simulink model "SUB_IoControl"  (R2018b)
settings: Solver=VariableStepDiscrete  StartTime=0.0  StopTime=10  RelTol=1e-3
PreLoadFcn:
  | if(exist('MBDS_ModelCallback', 'file'))
  |    MBDS_ModelCallback('PreLoad');
  | end
PostLoadFcn:
  | if(exist('MBDS_ModelCallback', 'file'))
  |    MBDS_ModelCallback('PostLoad');
  | end
InitFcn:
  | if(exist('MBDS_ModelCallback', 'file'))
  |    MBDS_ModelCallback('Init');
  | end
StartFcn:
  | if(exist('MBDS_ModelCallback', 'file'))
  |    MBDS_ModelCallback('Start');
  | end
StopFcn:
  | if(exist('MBDS_ModelCallback', 'file'))
  |    MBDS_ModelCallback('Stop');
  | end
undefined symbols (not defined in the file): sigbuilder_block
libraries: KIBES_Signal x742, MBDS_Modules x38, simulink x1
(part 8 of 8)

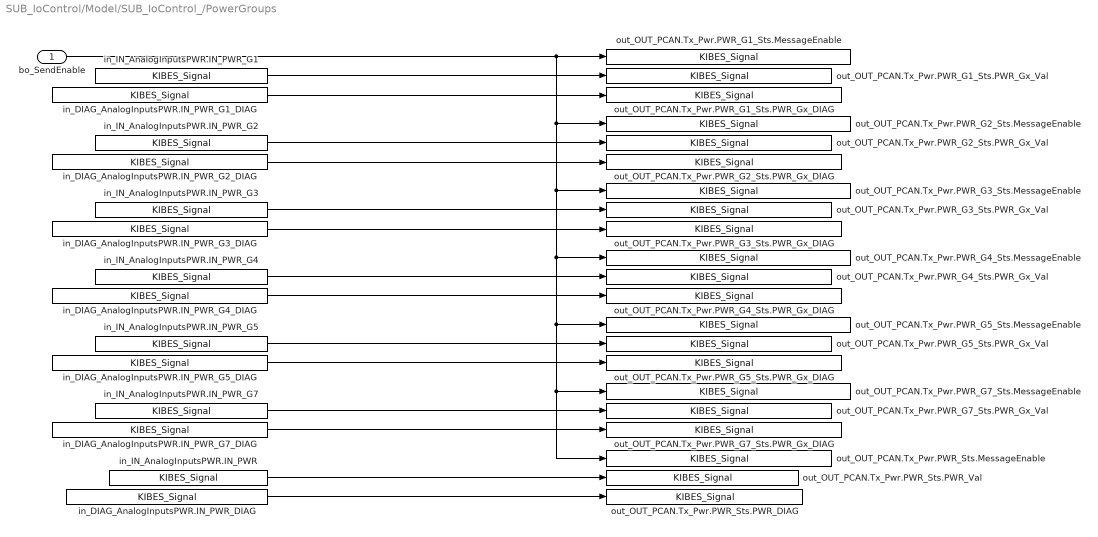
== system SUB_IoControl/Model/SUB_IoControl_/PowerGroups ==
  bo_SendEnable : Inport
  in_DIAG_AnalogInputsPWR.IN_PWR_DIAG : KIBES_Signal/KIBES_Signal  MBDS_LibraryBlock=on  DatabaseKey=722  SignalName=DIAG_AnalogInputsPWR.IN_PWR_DIAG  SymbolName=DIAG_AnalogInputsPWR_IN_PWR_DIAG_000722  DataType=uint16  Init=1  Slope=1  Bias=0  DataSize=1  fpDataType=uint16  BlockIOType=Inport  DeviceType=0
  in_DIAG_AnalogInputsPWR.IN_PWR_G1_DIAG : KIBES_Signal/KIBES_Signal  MBDS_LibraryBlock=on  DatabaseKey=724  SignalName=DIAG_AnalogInputsPWR.IN_PWR_G1_DIAG  SymbolName=DIAG_AnalogInputsPWR_IN_PWR_G1_DIAG_000724  DataType=uint16  Init=1  Slope=1  Bias=0  DataSize=1  fpDataType=uint16  BlockIOType=Inport  DeviceType=0
  in_DIAG_AnalogInputsPWR.IN_PWR_G2_DIAG : KIBES_Signal/KIBES_Signal  MBDS_LibraryBlock=on  DatabaseKey=726  SignalName=DIAG_AnalogInputsPWR.IN_PWR_G2_DIAG  SymbolName=DIAG_AnalogInputsPWR_IN_PWR_G2_DIAG_000726  DataType=uint16  Init=1  Slope=1  Bias=0  DataSize=1  fpDataType=uint16  BlockIOType=Inport  DeviceType=0
  in_DIAG_AnalogInputsPWR.IN_PWR_G3_DIAG : KIBES_Signal/KIBES_Signal  MBDS_LibraryBlock=on  DatabaseKey=734  SignalName=DIAG_AnalogInputsPWR.IN_PWR_G3_DIAG  SymbolName=DIAG_AnalogInputsPWR_IN_PWR_G3_DIAG_000734  DataType=uint16  Init=1  Slope=1  Bias=0  DataSize=1  fpDataType=uint16  BlockIOType=Inport  DeviceType=0
  in_DIAG_AnalogInputsPWR.IN_PWR_G4_DIAG : KIBES_Signal/KIBES_Signal  MBDS_LibraryBlock=on  DatabaseKey=728  SignalName=DIAG_AnalogInputsPWR.IN_PWR_G4_DIAG  SymbolName=DIAG_AnalogInputsPWR_IN_PWR_G4_DIAG_000728  DataType=uint16  Init=1  Slope=1  Bias=0  DataSize=1  fpDataType=uint16  BlockIOType=Inport  DeviceType=0
  in_DIAG_AnalogInputsPWR.IN_PWR_G5_DIAG : KIBES_Signal/KIBES_Signal  MBDS_LibraryBlock=on  DatabaseKey=730  SignalName=DIAG_AnalogInputsPWR.IN_PWR_G5_DIAG  SymbolName=DIAG_AnalogInputsPWR_IN_PWR_G5_DIAG_000730  DataType=uint16  Init=1  Slope=1  Bias=0  DataSize=1  fpDataType=uint16  BlockIOType=Inport  DeviceType=0
  in_DIAG_AnalogInputsPWR.IN_PWR_G7_DIAG : KIBES_Signal/KIBES_Signal  MBDS_LibraryBlock=on  DatabaseKey=732  SignalName=DIAG_AnalogInputsPWR.IN_PWR_G7_DIAG  SymbolName=DIAG_AnalogInputsPWR_IN_PWR_G7_DIAG_000732  DataType=uint16  Init=1  Slope=1  Bias=0  DataSize=1  fpDataType=uint16  BlockIOType=Inport  DeviceType=0
  in_IN_AnalogInputsPWR.IN_PWR : KIBES_Signal/KIBES_Signal  MBDS_LibraryBlock=on  DatabaseKey=721  SignalName=IN_AnalogInputsPWR.IN_PWR  SymbolName=IN_AnalogInputsPWR_IN_PWR_000721  DataType=uint32  Init=0  Slope=1  Bias=0  DataSize=1  fpDataType=uint32  BlockIOType=Inport  DeviceType=0
  in_IN_AnalogInputsPWR.IN_PWR_G1 : KIBES_Signal/KIBES_Signal  MBDS_LibraryBlock=on  DatabaseKey=723  SignalName=IN_AnalogInputsPWR.IN_PWR_G1  SymbolName=IN_AnalogInputsPWR_IN_PWR_G1_000723  DataType=uint16  Init=0  Slope=1  Bias=0  DataSize=1  fpDataType=uint16  BlockIOType=Inport  DeviceType=0
  in_IN_AnalogInputsPWR.IN_PWR_G2 : KIBES_Signal/KIBES_Signal  MBDS_LibraryBlock=on  DatabaseKey=725  SignalName=IN_AnalogInputsPWR.IN_PWR_G2  SymbolName=IN_AnalogInputsPWR_IN_PWR_G2_000725  DataType=uint16  Init=0  Slope=1  Bias=0  DataSize=1  fpDataType=uint16  BlockIOType=Inport  DeviceType=0
  in_IN_AnalogInputsPWR.IN_PWR_G3 : KIBES_Signal/KIBES_Signal  MBDS_LibraryBlock=on  DatabaseKey=733  SignalName=IN_AnalogInputsPWR.IN_PWR_G3  SymbolName=IN_AnalogInputsPWR_IN_PWR_G3_000733  DataType=uint16  Init=0  Slope=1  Bias=0  DataSize=1  fpDataType=uint16  BlockIOType=Inport  DeviceType=0
  in_IN_AnalogInputsPWR.IN_PWR_G4 : KIBES_Signal/KIBES_Signal  MBDS_LibraryBlock=on  DatabaseKey=727  SignalName=IN_AnalogInputsPWR.IN_PWR_G4  SymbolName=IN_AnalogInputsPWR_IN_PWR_G4_000727  DataType=uint16  Init=0  Slope=1  Bias=0  DataSize=1  fpDataType=uint16  BlockIOType=Inport  DeviceType=0
  in_IN_AnalogInputsPWR.IN_PWR_G5 : KIBES_Signal/KIBES_Signal  MBDS_LibraryBlock=on  DatabaseKey=729  SignalName=IN_AnalogInputsPWR.IN_PWR_G5  SymbolName=IN_AnalogInputsPWR_IN_PWR_G5_000729  DataType=uint16  Init=0  Slope=1  Bias=0  DataSize=1  fpDataType=uint16  BlockIOType=Inport  DeviceType=0
  in_IN_AnalogInputsPWR.IN_PWR_G7 : KIBES_Signal/KIBES_Signal  MBDS_LibraryBlock=on  DatabaseKey=731  SignalName=IN_AnalogInputsPWR.IN_PWR_G7  SymbolName=IN_AnalogInputsPWR_IN_PWR_G7_000731  DataType=uint16  Init=0  Slope=1  Bias=0  DataSize=1  fpDataType=uint16  BlockIOType=Inport  DeviceType=0
  out_OUT_PCAN.Tx_Pwr.PWR_G1_Sts.MessageEnable : KIBES_Signal/KIBES_Signal  MBDS_LibraryBlock=on  DatabaseKey=1777  SignalName=OUT_PCAN.Tx_Pwr.PWR_G1_Sts.MessageEnable  SymbolName=OUT_PCAN_Tx_Pwr_PWR_G1_Sts_MessageEnable_001777  DataType=boolean  Init=0  Slope=1  Bias=0  DataSize=1  fpDataType=boolean  BlockIOType=Outport  DeviceType=0
  out_OUT_PCAN.Tx_Pwr.PWR_G1_Sts.PWR_Gx_DIAG : KIBES_Signal/KIBES_Signal  MBDS_LibraryBlock=on  DatabaseKey=1763  SignalName=OUT_PCAN.Tx_Pwr.PWR_G1_Sts.PWR_Gx_DIAG  SymbolName=OUT_PCAN_Tx_Pwr_PWR_G1_Sts_PWR_Gx_DIAG_001763  DataType=uint16  Init=0  Slope=1  Bias=0  DataSize=1  fpDataType=uint16  BlockIOType=Outport  DeviceType=0
  out_OUT_PCAN.Tx_Pwr.PWR_G1_Sts.PWR_Gx_Val : KIBES_Signal/KIBES_Signal  MBDS_LibraryBlock=on  DatabaseKey=1764  SignalName=OUT_PCAN.Tx_Pwr.PWR_G1_Sts.PWR_Gx_Val  SymbolName=OUT_PCAN_Tx_Pwr_PWR_G1_Sts_PWR_Gx_Val_001764  DataType=uint16  Init=0  Slope=1  Bias=0  DataSize=1  fpDataType=uint16  BlockIOType=Outport  DeviceType=0
  out_OUT_PCAN.Tx_Pwr.PWR_G2_Sts.MessageEnable : KIBES_Signal/KIBES_Signal  MBDS_LibraryBlock=on  DatabaseKey=1778  SignalName=OUT_PCAN.Tx_Pwr.PWR_G2_Sts.MessageEnable  SymbolName=OUT_PCAN_Tx_Pwr_PWR_G2_Sts_MessageEnable_001778  DataType=boolean  Init=0  Slope=1  Bias=0  DataSize=1  fpDataType=boolean  BlockIOType=Outport  DeviceType=0
  out_OUT_PCAN.Tx_Pwr.PWR_G2_Sts.PWR_Gx_DIAG : KIBES_Signal/KIBES_Signal  MBDS_LibraryBlock=on  DatabaseKey=1765  SignalName=OUT_PCAN.Tx_Pwr.PWR_G2_Sts.PWR_Gx_DIAG  SymbolName=OUT_PCAN_Tx_Pwr_PWR_G2_Sts_PWR_Gx_DIAG_001765  DataType=uint16  Init=0  Slope=1  Bias=0  DataSize=1  fpDataType=uint16  BlockIOType=Outport  DeviceType=0
  out_OUT_PCAN.Tx_Pwr.PWR_G2_Sts.PWR_Gx_Val : KIBES_Signal/KIBES_Signal  MBDS_LibraryBlock=on  DatabaseKey=1766  SignalName=OUT_PCAN.Tx_Pwr.PWR_G2_Sts.PWR_Gx_Val  SymbolName=OUT_PCAN_Tx_Pwr_PWR_G2_Sts_PWR_Gx_Val_001766  DataType=uint16  Init=0  Slope=1  Bias=0  DataSize=1  fpDataType=uint16  BlockIOType=Outport  DeviceType=0
  out_OUT_PCAN.Tx_Pwr.PWR_G3_Sts.MessageEnable : KIBES_Signal/KIBES_Signal  MBDS_LibraryBlock=on  DatabaseKey=1779  SignalName=OUT_PCAN.Tx_Pwr.PWR_G3_Sts.MessageEnable  SymbolName=OUT_PCAN_Tx_Pwr_PWR_G3_Sts_MessageEnable_001779  DataType=boolean  Init=0  Slope=1  Bias=0  DataSize=1  fpDataType=boolean  BlockIOType=Outport  DeviceType=0
  out_OUT_PCAN.Tx_Pwr.PWR_G3_Sts.PWR_Gx_DIAG : KIBES_Signal/KIBES_Signal  MBDS_LibraryBlock=on  DatabaseKey=1767  SignalName=OUT_PCAN.Tx_Pwr.PWR_G3_Sts.PWR_Gx_DIAG  SymbolName=OUT_PCAN_Tx_Pwr_PWR_G3_Sts_PWR_Gx_DIAG_001767  DataType=uint16  Init=0  Slope=1  Bias=0  DataSize=1  fpDataType=uint16  BlockIOType=Outport  DeviceType=0
  out_OUT_PCAN.Tx_Pwr.PWR_G3_Sts.PWR_Gx_Val : KIBES_Signal/KIBES_Signal  MBDS_LibraryBlock=on  DatabaseKey=1768  SignalName=OUT_PCAN.Tx_Pwr.PWR_G3_Sts.PWR_Gx_Val  SymbolName=OUT_PCAN_Tx_Pwr_PWR_G3_Sts_PWR_Gx_Val_001768  DataType=uint16  Init=0  Slope=1  Bias=0  DataSize=1  fpDataType=uint16  BlockIOType=Outport  DeviceType=0
  out_OUT_PCAN.Tx_Pwr.PWR_G4_Sts.MessageEnable : KIBES_Signal/KIBES_Signal  MBDS_LibraryBlock=on  DatabaseKey=1780  SignalName=OUT_PCAN.Tx_Pwr.PWR_G4_Sts.MessageEnable  SymbolName=OUT_PCAN_Tx_Pwr_PWR_G4_Sts_MessageEnable_001780  DataType=boolean  Init=0  Slope=1  Bias=0  DataSize=1  fpDataType=boolean  BlockIOType=Outport  DeviceType=0
  out_OUT_PCAN.Tx_Pwr.PWR_G4_Sts.PWR_Gx_DIAG : KIBES_Signal/KIBES_Signal  MBDS_LibraryBlock=on  DatabaseKey=1769  SignalName=OUT_PCAN.Tx_Pwr.PWR_G4_Sts.PWR_Gx_DIAG  SymbolName=OUT_PCAN_Tx_Pwr_PWR_G4_Sts_PWR_Gx_DIAG_001769  DataType=uint16  Init=0  Slope=1  Bias=0  DataSize=1  fpDataType=uint16  BlockIOType=Outport  DeviceType=0
  out_OUT_PCAN.Tx_Pwr.PWR_G4_Sts.PWR_Gx_Val : KIBES_Signal/KIBES_Signal  MBDS_LibraryBlock=on  DatabaseKey=1770  SignalName=OUT_PCAN.Tx_Pwr.PWR_G4_Sts.PWR_Gx_Val  SymbolName=OUT_PCAN_Tx_Pwr_PWR_G4_Sts_PWR_Gx_Val_001770  DataType=uint16  Init=0  Slope=1  Bias=0  DataSize=1  fpDataType=uint16  BlockIOType=Outport  DeviceType=0
  out_OUT_PCAN.Tx_Pwr.PWR_G5_Sts.MessageEnable : KIBES_Signal/KIBES_Signal  MBDS_LibraryBlock=on  DatabaseKey=1781  SignalName=OUT_PCAN.Tx_Pwr.PWR_G5_Sts.MessageEnable  SymbolName=OUT_PCAN_Tx_Pwr_PWR_G5_Sts_MessageEnable_001781  DataType=boolean  Init=0  Slope=1  Bias=0  DataSize=1  fpDataType=boolean  BlockIOType=Outport  DeviceType=0
  out_OUT_PCAN.Tx_Pwr.PWR_G5_Sts.PWR_Gx_DIAG : KIBES_Signal/KIBES_Signal  MBDS_LibraryBlock=on  DatabaseKey=1771  SignalName=OUT_PCAN.Tx_Pwr.PWR_G5_Sts.PWR_Gx_DIAG  SymbolName=OUT_PCAN_Tx_Pwr_PWR_G5_Sts_PWR_Gx_DIAG_001771  DataType=uint16  Init=0  Slope=1  Bias=0  DataSize=1  fpDataType=uint16  BlockIOType=Outport  DeviceType=0
  out_OUT_PCAN.Tx_Pwr.PWR_G5_Sts.PWR_Gx_Val : KIBES_Signal/KIBES_Signal  MBDS_LibraryBlock=on  DatabaseKey=1772  SignalName=OUT_PCAN.Tx_Pwr.PWR_G5_Sts.PWR_Gx_Val  SymbolName=OUT_PCAN_Tx_Pwr_PWR_G5_Sts_PWR_Gx_Val_001772  DataType=uint16  Init=0  Slope=1  Bias=0  DataSize=1  fpDataType=uint16  BlockIOType=Outport  DeviceType=0
  out_OUT_PCAN.Tx_Pwr.PWR_G7_Sts.MessageEnable : KIBES_Signal/KIBES_Signal  MBDS_LibraryBlock=on  DatabaseKey=1782  SignalName=OUT_PCAN.Tx_Pwr.PWR_G7_Sts.MessageEnable  SymbolName=OUT_PCAN_Tx_Pwr_PWR_G7_Sts_MessageEnable_001782  DataType=boolean  Init=0  Slope=1  Bias=0  DataSize=1  fpDataType=boolean  BlockIOType=Outport  DeviceType=0
  out_OUT_PCAN.Tx_Pwr.PWR_G7_Sts.PWR_Gx_DIAG : KIBES_Signal/KIBES_Signal  MBDS_LibraryBlock=on  DatabaseKey=1773  SignalName=OUT_PCAN.Tx_Pwr.PWR_G7_Sts.PWR_Gx_DIAG  SymbolName=OUT_PCAN_Tx_Pwr_PWR_G7_Sts_PWR_Gx_DIAG_001773  DataType=uint16  Init=0  Slope=1  Bias=0  DataSize=1  fpDataType=uint16  BlockIOType=Outport  DeviceType=0
  out_OUT_PCAN.Tx_Pwr.PWR_G7_Sts.PWR_Gx_Val : KIBES_Signal/KIBES_Signal  MBDS_LibraryBlock=on  DatabaseKey=1774  SignalName=OUT_PCAN.Tx_Pwr.PWR_G7_Sts.PWR_Gx_Val  SymbolName=OUT_PCAN_Tx_Pwr_PWR_G7_Sts_PWR_Gx_Val_001774  DataType=uint16  Init=0  Slope=1  Bias=0  DataSize=1  fpDataType=uint16  BlockIOType=Outport  DeviceType=0
  out_OUT_PCAN.Tx_Pwr.PWR_Sts.MessageEnable : KIBES_Signal/KIBES_Signal  MBDS_LibraryBlock=on  DatabaseKey=1783  SignalName=OUT_PCAN.Tx_Pwr.PWR_Sts.MessageEnable  SymbolName=OUT_PCAN_Tx_Pwr_PWR_Sts_MessageEnable_001783  DataType=boolean  Init=0  Slope=1  Bias=0  DataSize=1  fpDataType=boolean  BlockIOType=Outport  DeviceType=0
  out_OUT_PCAN.Tx_Pwr.PWR_Sts.PWR_DIAG : KIBES_Signal/KIBES_Signal  MBDS_LibraryBlock=on  DatabaseKey=1775  SignalName=OUT_PCAN.Tx_Pwr.PWR_Sts.PWR_DIAG  SymbolName=OUT_PCAN_Tx_Pwr_PWR_Sts_PWR_DIAG_001775  DataType=uint16  Init=0  Slope=1  Bias=0  DataSize=1  fpDataType=uint16  BlockIOType=Outport  DeviceType=0
  out_OUT_PCAN.Tx_Pwr.PWR_Sts.PWR_Val : KIBES_Signal/KIBES_Signal  MBDS_LibraryBlock=on  DatabaseKey=1776  SignalName=OUT_PCAN.Tx_Pwr.PWR_Sts.PWR_Val  SymbolName=OUT_PCAN_Tx_Pwr_PWR_Sts_PWR_Val_001776  DataType=uint32  Init=0  Slope=1  Bias=0  DataSize=1  fpDataType=uint32  BlockIOType=Outport  DeviceType=0
  wires:
  in_IN_AnalogInputsPWR.IN_PWR_G2/1 -> out_OUT_PCAN.Tx_Pwr.PWR_G2_Sts.PWR_Gx_Val/1
  in_IN_AnalogInputsPWR.IN_PWR_G1/1 -> out_OUT_PCAN.Tx_Pwr.PWR_G1_Sts.PWR_Gx_Val/1
  in_IN_AnalogInputsPWR.IN_PWR_G5/1 -> out_OUT_PCAN.Tx_Pwr.PWR_G5_Sts.PWR_Gx_Val/1
  bo_SendEnable/1 -> out_OUT_PCAN.Tx_Pwr.PWR_G1_Sts.MessageEnable/1, out_OUT_PCAN.Tx_Pwr.PWR_G2_Sts.MessageEnable/1, out_OUT_PCAN.Tx_Pwr.PWR_G3_Sts.MessageEnable/1, out_OUT_PCAN.Tx_Pwr.PWR_G4_Sts.MessageEnable/1, out_OUT_PCAN.Tx_Pwr.PWR_G5_Sts.MessageEnable/1, out_OUT_PCAN.Tx_Pwr.PWR_Sts.MessageEnable/1, out_OUT_PCAN.Tx_Pwr.PWR_G7_Sts.MessageEnable/1
  in_IN_AnalogInputsPWR.IN_PWR_G4/1 -> out_OUT_PCAN.Tx_Pwr.PWR_G4_Sts.PWR_Gx_Val/1
  in_DIAG_AnalogInputsPWR.IN_PWR_G1_DIAG/1 -> out_OUT_PCAN.Tx_Pwr.PWR_G1_Sts.PWR_Gx_DIAG/1
  in_DIAG_AnalogInputsPWR.IN_PWR_DIAG/1 -> out_OUT_PCAN.Tx_Pwr.PWR_Sts.PWR_DIAG/1
  in_IN_AnalogInputsPWR.IN_PWR/1 -> out_OUT_PCAN.Tx_Pwr.PWR_Sts.PWR_Val/1
  in_DIAG_AnalogInputsPWR.IN_PWR_G2_DIAG/1 -> out_OUT_PCAN.Tx_Pwr.PWR_G2_Sts.PWR_Gx_DIAG/1
  in_DIAG_AnalogInputsPWR.IN_PWR_G5_DIAG/1 -> out_OUT_PCAN.Tx_Pwr.PWR_G5_Sts.PWR_Gx_DIAG/1
  in_DIAG_AnalogInputsPWR.IN_PWR_G7_DIAG/1 -> out_OUT_PCAN.Tx_Pwr.PWR_G7_Sts.PWR_Gx_DIAG/1
  in_IN_AnalogInputsPWR.IN_PWR_G3/1 -> out_OUT_PCAN.Tx_Pwr.PWR_G3_Sts.PWR_Gx_Val/1
  in_IN_AnalogInputsPWR.IN_PWR_G7/1 -> out_OUT_PCAN.Tx_Pwr.PWR_G7_Sts.PWR_Gx_Val/1
  in_DIAG_AnalogInputsPWR.IN_PWR_G4_DIAG/1 -> out_OUT_PCAN.Tx_Pwr.PWR_G4_Sts.PWR_Gx_DIAG/1
  in_DIAG_AnalogInputsPWR.IN_PWR_G3_DIAG/1 -> out_OUT_PCAN.Tx_Pwr.PWR_G3_Sts.PWR_Gx_DIAG/1

== system SUB_IoControl/Outputs/AnalyseOutputs/And ==
  note: AND
  u1 : Inport  OutDataTypeStr=boolean
  u2 : Inport  Port=2  OutDataTypeStr=boolean
  DataType : DataTypeConversion  OutDataTypeStr=boolean
  Operator : Logic  AllPortsSameDT=off  OutDataTypeStr=boolean
  y : Outport
  wires:
  Operator/1 -> DataType/1
  u1/1 -> Operator/1
  u2/1 -> Operator/2
  DataType/1 -> y/1

== system SUB_IoControl/Outputs/AnalyseOutputs/LE1 ==
  note: LE
  u1 : Inport
  u2 : Inport  Port=2
  Operator : RelationalOperator  Operator=<=  OutDataTypeStr=boolean  RndMeth=Nearest  InputSameDT=on
  y : Outport
  wires:
  Operator/1 -> y/1
  u2/1 -> Operator/2
  u1/1 -> Operator/1

== system SUB_IoControl/Outputs/AnalyseOutputs/LE2 ==
  note: LE
  u1 : Inport
  u2 : Inport  Port=2
  Operator : RelationalOperator  Operator=<=  OutDataTypeStr=boolean  RndMeth=Nearest  InputSameDT=on
  y : Outport
  wires:
  Operator/1 -> y/1
  u2/1 -> Operator/2
  u1/1 -> Operator/1

== system SUB_IoControl/Model/SUB_IoControl_/AnalogInputs/AND ==
  note: AND
  u1 : Inport  OutDataTypeStr=boolean
  u2 : Inport  Port=2  OutDataTypeStr=boolean
  DataType : DataTypeConversion  OutDataTypeStr=boolean
  Operator : Logic  AllPortsSameDT=off  OutDataTypeStr=boolean
  y : Outport
  wires:
  Operator/1 -> DataType/1
  u1/1 -> Operator/1
  u2/1 -> Operator/2
  DataType/1 -> y/1

== system SUB_IoControl/Model/SUB_IoControl_/AnalogInputs/AND1 ==
  note: AND
  u1 : Inport  OutDataTypeStr=boolean
  u2 : Inport  Port=2  OutDataTypeStr=boolean
  DataType : DataTypeConversion  OutDataTypeStr=boolean
  Operator : Logic  AllPortsSameDT=off  OutDataTypeStr=boolean
  y : Outport
  wires:
  Operator/1 -> DataType/1
  u1/1 -> Operator/1
  u2/1 -> Operator/2
  DataType/1 -> y/1

== system SUB_IoControl/Model/SUB_IoControl_/AnalogInputs/AND2 ==
  note: AND
  u1 : Inport  OutDataTypeStr=boolean
  u2 : Inport  Port=2  OutDataTypeStr=boolean
  DataType : DataTypeConversion  OutDataTypeStr=boolean
  Operator : Logic  AllPortsSameDT=off  OutDataTypeStr=boolean
  y : Outport
  wires:
  Operator/1 -> DataType/1
  u1/1 -> Operator/1
  u2/1 -> Operator/2
  DataType/1 -> y/1

== system SUB_IoControl/Model/SUB_IoControl_/AnalogInputs/AND3 ==
  note: AND
  u1 : Inport  OutDataTypeStr=boolean
  u2 : Inport  Port=2  OutDataTypeStr=boolean
  DataType : DataTypeConversion  OutDataTypeStr=boolean
  Operator : Logic  AllPortsSameDT=off  OutDataTypeStr=boolean
  y : Outport
  wires:
  Operator/1 -> DataType/1
  u1/1 -> Operator/1
  u2/1 -> Operator/2
  DataType/1 -> y/1

== system SUB_IoControl/Model/SUB_IoControl_/AnalogInputs/EQ ==
  note: EQ
  u1 : Inport
  u2 : Inport  Port=2
  Operator : RelationalOperator  Operator===  OutDataTypeStr=boolean  RndMeth=Nearest  InputSameDT=on
  y : Outport
  wires:
  Operator/1 -> y/1
  u1/1 -> Operator/1
  u2/1 -> Operator/2

== system SUB_IoControl/Model/SUB_IoControl_/AnalogsSupply/AND ==
  note: AND
  u1 : Inport  OutDataTypeStr=boolean
  u2 : Inport  Port=2  OutDataTypeStr=boolean
  DataType : DataTypeConversion  OutDataTypeStr=boolean
  Operator : Logic  AllPortsSameDT=off  OutDataTypeStr=boolean
  y : Outport
  wires:
  Operator/1 -> DataType/1
  u1/1 -> Operator/1
  u2/1 -> Operator/2
  DataType/1 -> y/1

== system SUB_IoControl/Model/SUB_IoControl_/AnalogsSupply/AND1 ==
  note: AND
  u1 : Inport  OutDataTypeStr=boolean
  u2 : Inport  Port=2  OutDataTypeStr=boolean
  DataType : DataTypeConversion  OutDataTypeStr=boolean
  Operator : Logic  AllPortsSameDT=off  OutDataTypeStr=boolean
  y : Outport
  wires:
  Operator/1 -> DataType/1
  u1/1 -> Operator/1
  u2/1 -> Operator/2
  DataType/1 -> y/1

== system SUB_IoControl/Model/SUB_IoControl_/AnalogsSupply/AND2 ==
  note: AND
  u1 : Inport  OutDataTypeStr=boolean
  u2 : Inport  Port=2  OutDataTypeStr=boolean
  DataType : DataTypeConversion  OutDataTypeStr=boolean
  Operator : Logic  AllPortsSameDT=off  OutDataTypeStr=boolean
  y : Outport
  wires:
  Operator/1 -> DataType/1
  u1/1 -> Operator/1
  u2/1 -> Operator/2
  DataType/1 -> y/1

== system SUB_IoControl/Model/SUB_IoControl_/AnalogsSupply/EQ ==
  note: EQ
  u1 : Inport
  u2 : Inport  Port=2
  Operator : RelationalOperator  Operator===  OutDataTypeStr=boolean  RndMeth=Nearest  InputSameDT=on
  y : Outport
  wires:
  Operator/1 -> y/1
  u1/1 -> Operator/1
  u2/1 -> Operator/2

== system SUB_IoControl/Model/SUB_IoControl_/DigitalOutputs/AND1 ==
  note: AND
  u1 : Inport  OutDataTypeStr=boolean
  u2 : Inport  Port=2  OutDataTypeStr=boolean
  DataType : DataTypeConversion  OutDataTypeStr=boolean
  Operator : Logic  AllPortsSameDT=off  OutDataTypeStr=boolean
  y : Outport
  wires:
  Operator/1 -> DataType/1
  u1/1 -> Operator/1
  u2/1 -> Operator/2
  DataType/1 -> y/1

== system SUB_IoControl/Model/SUB_IoControl_/DigitalOutputs/AND10 ==
  note: AND
  u1 : Inport  OutDataTypeStr=boolean
  u2 : Inport  Port=2  OutDataTypeStr=boolean
  DataType : DataTypeConversion  OutDataTypeStr=boolean
  Operator : Logic  AllPortsSameDT=off  OutDataTypeStr=boolean
  y : Outport
  wires:
  Operator/1 -> DataType/1
  u1/1 -> Operator/1
  u2/1 -> Operator/2
  DataType/1 -> y/1

== system SUB_IoControl/Model/SUB_IoControl_/DigitalOutputs/AND11 ==
  note: AND
  u1 : Inport  OutDataTypeStr=boolean
  u2 : Inport  Port=2  OutDataTypeStr=boolean
  DataType : DataTypeConversion  OutDataTypeStr=boolean
  Operator : Logic  AllPortsSameDT=off  OutDataTypeStr=boolean
  y : Outport
  wires:
  Operator/1 -> DataType/1
  u1/1 -> Operator/1
  u2/1 -> Operator/2
  DataType/1 -> y/1

== system SUB_IoControl/Model/SUB_IoControl_/DigitalOutputs/AND12 ==
  note: AND
  u1 : Inport  OutDataTypeStr=boolean
  u2 : Inport  Port=2  OutDataTypeStr=boolean
  DataType : DataTypeConversion  OutDataTypeStr=boolean
  Operator : Logic  AllPortsSameDT=off  OutDataTypeStr=boolean
  y : Outport
  wires:
  Operator/1 -> DataType/1
  u1/1 -> Operator/1
  u2/1 -> Operator/2
  DataType/1 -> y/1

== system SUB_IoControl/Model/SUB_IoControl_/DigitalOutputs/AND13 ==
  note: AND
  u1 : Inport  OutDataTypeStr=boolean
  u2 : Inport  Port=2  OutDataTypeStr=boolean
  DataType : DataTypeConversion  OutDataTypeStr=boolean
  Operator : Logic  AllPortsSameDT=off  OutDataTypeStr=boolean
  y : Outport
  wires:
  Operator/1 -> DataType/1
  u1/1 -> Operator/1
  u2/1 -> Operator/2
  DataType/1 -> y/1

== system SUB_IoControl/Model/SUB_IoControl_/DigitalOutputs/AND14 ==
  note: AND
  u1 : Inport  OutDataTypeStr=boolean
  u2 : Inport  Port=2  OutDataTypeStr=boolean
  DataType : DataTypeConversion  OutDataTypeStr=boolean
  Operator : Logic  AllPortsSameDT=off  OutDataTypeStr=boolean
  y : Outport
  wires:
  Operator/1 -> DataType/1
  u1/1 -> Operator/1
  u2/1 -> Operator/2
  DataType/1 -> y/1

== system SUB_IoControl/Model/SUB_IoControl_/DigitalOutputs/AND15 ==
  note: AND
  u1 : Inport  OutDataTypeStr=boolean
  u2 : Inport  Port=2  OutDataTypeStr=boolean
  DataType : DataTypeConversion  OutDataTypeStr=boolean
  Operator : Logic  AllPortsSameDT=off  OutDataTypeStr=boolean
  y : Outport
  wires:
  Operator/1 -> DataType/1
  u1/1 -> Operator/1
  u2/1 -> Operator/2
  DataType/1 -> y/1

== system SUB_IoControl/Model/SUB_IoControl_/DigitalOutputs/AND16 ==
  note: AND
  u1 : Inport  OutDataTypeStr=boolean
  u2 : Inport  Port=2  OutDataTypeStr=boolean
  DataType : DataTypeConversion  OutDataTypeStr=boolean
  Operator : Logic  AllPortsSameDT=off  OutDataTypeStr=boolean
  y : Outport
  wires:
  Operator/1 -> DataType/1
  u1/1 -> Operator/1
  u2/1 -> Operator/2
  DataType/1 -> y/1

== system SUB_IoControl/Model/SUB_IoControl_/DigitalOutputs/AND17 ==
  note: AND
  u1 : Inport  OutDataTypeStr=boolean
  u2 : Inport  Port=2  OutDataTypeStr=boolean
  DataType : DataTypeConversion  OutDataTypeStr=boolean
  Operator : Logic  AllPortsSameDT=off  OutDataTypeStr=boolean
  y : Outport
  wires:
  Operator/1 -> DataType/1
  u1/1 -> Operator/1
  u2/1 -> Operator/2
  DataType/1 -> y/1

== system SUB_IoControl/Model/SUB_IoControl_/DigitalOutputs/AND18 ==
  note: AND
  u1 : Inport  OutDataTypeStr=boolean
  u2 : Inport  Port=2  OutDataTypeStr=boolean
  DataType : DataTypeConversion  OutDataTypeStr=boolean
  Operator : Logic  AllPortsSameDT=off  OutDataTypeStr=boolean
  y : Outport
  wires:
  Operator/1 -> DataType/1
  u1/1 -> Operator/1
  u2/1 -> Operator/2
  DataType/1 -> y/1

== system SUB_IoControl/Model/SUB_IoControl_/DigitalOutputs/EQ ==
  note: EQ
  u1 : Inport
  u2 : Inport  Port=2
  Operator : RelationalOperator  Operator===  OutDataTypeStr=boolean  RndMeth=Nearest  InputSameDT=on
  y : Outport
  wires:
  Operator/1 -> y/1
  u1/1 -> Operator/1
  u2/1 -> Operator/2

== system SUB_IoControl/Model/SUB_IoControl_/PWMs/AND ==
  note: AND
  u1 : Inport  OutDataTypeStr=boolean
  u2 : Inport  Port=2  OutDataTypeStr=boolean
  DataType : DataTypeConversion  OutDataTypeStr=boolean
  Operator : Logic  AllPortsSameDT=off  OutDataTypeStr=boolean
  y : Outport
  wires:
  Operator/1 -> DataType/1
  u1/1 -> Operator/1
  u2/1 -> Operator/2
  DataType/1 -> y/1

== system SUB_IoControl/Model/SUB_IoControl_/PWMs/AND1 ==
  note: AND
  u1 : Inport  OutDataTypeStr=boolean
  u2 : Inport  Port=2  OutDataTypeStr=boolean
  DataType : DataTypeConversion  OutDataTypeStr=boolean
  Operator : Logic  AllPortsSameDT=off  OutDataTypeStr=boolean
  y : Outport
  wires:
  Operator/1 -> DataType/1
  u1/1 -> Operator/1
  u2/1 -> Operator/2
  DataType/1 -> y/1

== system SUB_IoControl/Model/SUB_IoControl_/PWMs/EQ ==
  note: EQ
  u1 : Inport
  u2 : Inport  Port=2
  Operator : RelationalOperator  Operator===  OutDataTypeStr=boolean  RndMeth=Nearest  InputSameDT=on
  y : Outport
  wires:
  Operator/1 -> y/1
  u1/1 -> Operator/1
  u2/1 -> Operator/2

== system SUB_IoControl/Model/SUB_IoControl_/PWMs/EQ1 ==
  note: EQ
  u1 : Inport
  u2 : Inport  Port=2
  Operator : RelationalOperator  Operator===  OutDataTypeStr=boolean  RndMeth=Nearest  InputSameDT=on
  y : Outport
  wires:
  Operator/1 -> y/1
  u1/1 -> Operator/1
  u2/1 -> Operator/2

== system SUB_IoControl/Model/SUB_IoControl_/PWMs/GT ==
  note: GT
  u1 : Inport
  u2 : Inport  Port=2
  Operator : RelationalOperator  Operator=>  OutDataTypeStr=boolean  RndMeth=Nearest  InputSameDT=on
  y : Outport
  wires:
  u2/1 -> Operator/2
  u1/1 -> Operator/1
  Operator/1 -> y/1

== system SUB_IoControl/Model/SUB_IoControl_/PWMs/GT1 ==
  note: GT
  u1 : Inport
  u2 : Inport  Port=2
  Operator : RelationalOperator  Operator=>  OutDataTypeStr=boolean  RndMeth=Nearest  InputSameDT=on
  y : Outport
  wires:
  u2/1 -> Operator/2
  u1/1 -> Operator/1
  Operator/1 -> y/1

== system SUB_IoControl/Model/SUB_IoControl_/PWMs/GT2 ==
  note: GT
  u1 : Inport
  u2 : Inport  Port=2
  Operator : RelationalOperator  Operator=>  OutDataTypeStr=boolean  RndMeth=Nearest  InputSameDT=on
  y : Outport
  wires:
  u2/1 -> Operator/2
  u1/1 -> Operator/1
  Operator/1 -> y/1

== system SUB_IoControl/Model/SUB_IoControl_/PWMs/GT3 ==
  note: GT
  u1 : Inport
  u2 : Inport  Port=2
  Operator : RelationalOperator  Operator=>  OutDataTypeStr=boolean  RndMeth=Nearest  InputSameDT=on
  y : Outport
  wires:
  u2/1 -> Operator/2
  u1/1 -> Operator/1
  Operator/1 -> y/1

== system SUB_IoControl/Model/SUB_IoControl_/PWMs/GT4 ==
  note: GT
  u1 : Inport
  u2 : Inport  Port=2
  Operator : RelationalOperator  Operator=>  OutDataTypeStr=boolean  RndMeth=Nearest  InputSameDT=on
  y : Outport
  wires:
  u2/1 -> Operator/2
  u1/1 -> Operator/1
  Operator/1 -> y/1

== system SUB_IoControl/Model/SUB_IoControl_/PWMs/GT5 ==
  note: GT
  u1 : Inport
  u2 : Inport  Port=2
  Operator : RelationalOperator  Operator=>  OutDataTypeStr=boolean  RndMeth=Nearest  InputSameDT=on
  y : Outport
  wires:
  u2/1 -> Operator/2
  u1/1 -> Operator/1
  Operator/1 -> y/1

== system SUB_IoControl/Model/SUB_IoControl_/PWMs/GT6 ==
  note: GT
  u1 : Inport
  u2 : Inport  Port=2
  Operator : RelationalOperator  Operator=>  OutDataTypeStr=boolean  RndMeth=Nearest  InputSameDT=on
  y : Outport
  wires:
  u2/1 -> Operator/2
  u1/1 -> Operator/1
  Operator/1 -> y/1

== system SUB_IoControl/Model/SUB_IoControl_/PWMs/GT7 ==
  note: GT
  u1 : Inport
  u2 : Inport  Port=2
  Operator : RelationalOperator  Operator=>  OutDataTypeStr=boolean  RndMeth=Nearest  InputSameDT=on
  y : Outport
  wires:
  u2/1 -> Operator/2
  u1/1 -> Operator/1
  Operator/1 -> y/1

== system SUB_IoControl/Model/SUB_IoControl_/PWMs/GT8 ==
  note: GT
  u1 : Inport
  u2 : Inport  Port=2
  Operator : RelationalOperator  Operator=>  OutDataTypeStr=boolean  RndMeth=Nearest  InputSameDT=on
  y : Outport
  wires:
  u2/1 -> Operator/2
  u1/1 -> Operator/1
  Operator/1 -> y/1

== stateflow chart SUB_IoControl/Model/SUB_IoControl_/DigitalOutputs/BlinkSource ==
  state Blink_ON
    en:
    u16_Timer=uint16(1);
    bo_Blink = true;
    du:
    u16_Timer++;
  state Blink_OFF
    en:
    u16_Timer=uint16(1);
    bo_Blink = false;
    du:
    u16_Timer++;
  (default) -> Blink_ON
  Blink_OFF -> Blink_ON : [u16_Timer >= u16_PeriodTime]
  Blink_ON -> Blink_OFF : [u16_Timer >= u16_PeriodTime]
  data: u16_Timer local uint16 =0; bo_Blink output boolean =false; u16_PeriodTime input uint16 =12
